simulink subsystem "FTPiero"  (R2023b)
settings: Solver=VariableStepAuto  StartTime=0.0  StopTime=10.0  RelTol=1e-3
settings Model: Creator=Claudia Ada  LastModifiedBy=pablo

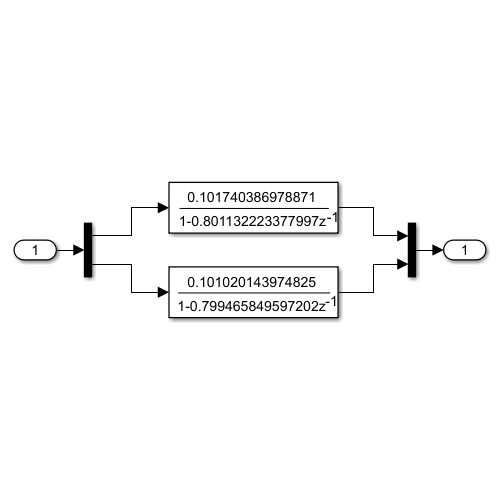
[thumbnail: Simulink's stored preview of the top-level diagram]
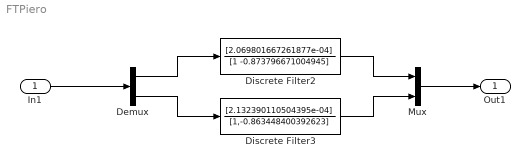
== system FTPiero ==
  In1 : Inport
  Demux : Demux  Outputs=2
  Discrete Filter2 : DiscreteFilter  Numerator=[2.069801667261877e-04]  Denominator=[1 -0.873796671004945]
  Discrete Filter3 : DiscreteFilter  Numerator=[2.132390110504395e-04]  Denominator=[1,-0.863448400392623]
  Mux : Mux  Inputs=2
  Out1 : Outport  OutDataTypeStr=double
  wires:
  Discrete Filter3/1 -> Mux/2
  Mux/1 -> Out1/1
  Demux/1 -> Discrete Filter2/1
  In1/1 -> Demux/1
  Discrete Filter2/1 -> Mux/1
  Demux/2 -> Discrete Filter3/1
